simulink model "Project2DigiCont"  (R2017b)
settings: Solver=VariableStepAuto  StartTime=0.0  StopTime=inf  RelTol=1e-3
libraries: Alarm_Library x1, Bump_SensorLib x1, Sensor_Wheellib x1
settings Model: Creator=segadiallo  LastModifiedBy=segadiallo

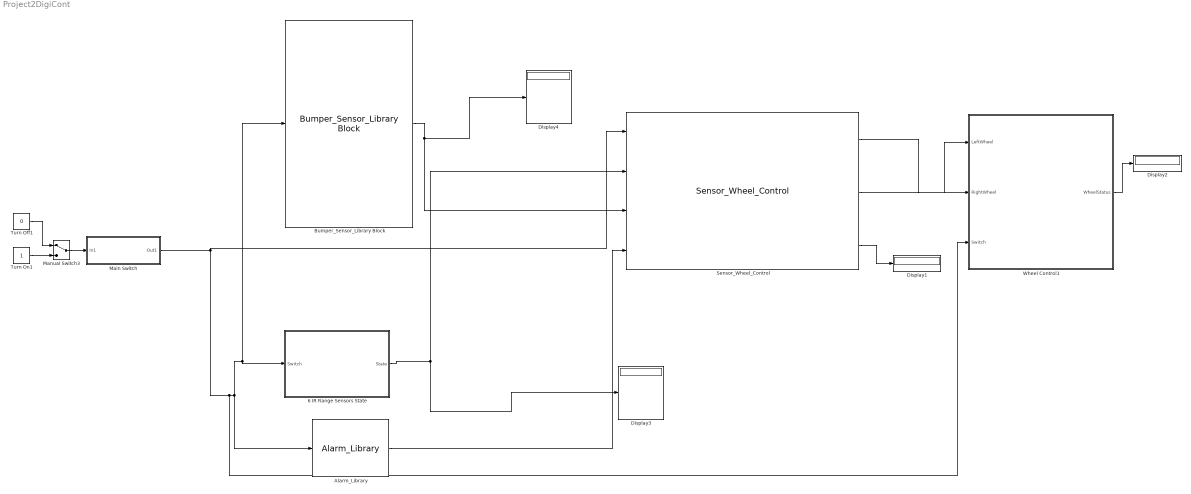
== system Project2DigiCont ==
  6 IR Range Sensors State : Subsystem  AncestorBlock=RoombaSimulink/6 IR Range Sensors State  mask(Sensor Read){}
      mask help:
      | Input 0 to turn off block
      | Input 1 to turn on block
      mask Display:
      | disp('IR Sensors State')
      | port_label('input',1,'Control')
      | port_label('output',1,'State')
  Alarm_Library : Alarm_Library/Alarm_Library  SystemSampleTime=-1
  Bumper_Sensor_Library Block : Bump_SensorLib/Bumper_Sensor_Library Block
  Display{1..4} (4 alike) : Display
  Main Switch : Subsystem
      mask Display:
      | disp('Main Switch')
      | port_label('output',1,'inputV')
      | port_label('input',1,'Go')
  Manual Switch3 : ManualSwitch
  Sensor_Wheel_Control : Sensor_Wheellib/Sensor_Wheel_Control  v0=0.2
  Turn Off1 : Constant  Value=0
  Turn On1 : Constant
  Wheel Control1 : Subsystem  AncestorBlock=RoombaSimulink/Wheel Control  mask(Control){}
      mask help:
      | Input -0.5~0.5 to LeftWheel and RightWheel to control the two wheels independently.
      | Switch: input 0 to turn off block; input 1 to turn on block; input 2 to pause wheel motions.
      mask Display:
      | disp('Wheel Control')
      | port_label('input',1,'LeftWheel')
      | port_label('input',2,'RightWheel')
      | port_label('input',3,'Control')
      | port_label('output',1,'Status')
      | %port_label('input',4,'Break')
  wires:
  Wheel Control1/1(WheelStatus) -> Display2/1
  6 IR Range Sensors State/1("State ") -> Display3/1, Sensor_Wheel_Control/2
  Turn Off1/1 -> Manual Switch3/1
  Turn On1/1 -> Manual Switch3/2
  Manual Switch3/1 -> Main Switch/1(In1)
  Main Switch/1(Out1) -> Wheel Control1/3(Switch), 6 IR Range Sensors State/1(Switch), Bumper_Sensor_Library Block/1, Alarm_Library/1, Sensor_Wheel_Control/1
  Sensor_Wheel_Control/1 -> Wheel Control1/2(RightWheel)
  Sensor_Wheel_Control/2 -> Wheel Control1/1(LeftWheel)
  Bumper_Sensor_Library Block/1 -> Display4/1, Sensor_Wheel_Control/3
  Sensor_Wheel_Control/3 -> Display1/1
  Alarm_Library/1 -> Sensor_Wheel_Control/4

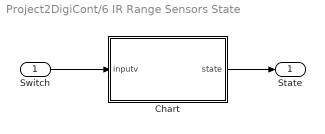
== system Project2DigiCont/6 IR Range Sensors State ==
  Switch : Inport
  Chart : Stateflow chart  TreatAsAtomicUnit=on
  "State " : Outport
  wires:
  Switch/1 -> Chart/1(inputv)
  Chart/1(state) -> "State "/1

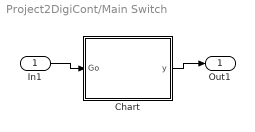
== system Project2DigiCont/Main Switch ==
  In1 : Inport
  Chart : Stateflow chart  TreatAsAtomicUnit=on
  Out1 : Outport
  wires:
  Chart/1(y) -> Out1/1
  In1/1 -> Chart/1(Go)

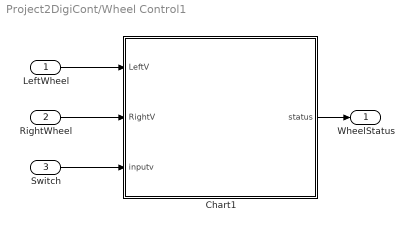
== system Project2DigiCont/Wheel Control1 ==
  LeftWheel : Inport
  RightWheel : Inport  Port=2
  Switch : Inport  Port=3
  Chart1 : Stateflow chart  TreatAsAtomicUnit=on
  WheelStatus : Outport
  wires:
  Switch/1 -> Chart1/3(inputv)
  RightWheel/1 -> Chart1/2(RightV)
  Chart1/1(status) -> WheelStatus/1
  LeftWheel/1 -> Chart1/1(LeftV)

== stateflow chart Project2DigiCont/Wheel Control1/Chart1 ==
  state START
    entry: status=0
  state Connect
    entry: coder.extrinsic('evalin')
    so=evalin('base','objWs')
  state Run
    entry,du:
    coder.extrinsic('SetWheelVelRoomba')
    SetWheelVelRoomba(so,RightV, LeftV)
    status=1
  state Off
    %entry: fclose(so);
    entry:  status=0
  state Pause [commented out]
    entry:
    coder.extrinsic('SetWheelVelRoomba')
    SetWheelVelRoomba(so,0, 0)
    status=2
  (default) -> START
  Off -> Connect : [inputv==4]
  START -> Connect : [inputv==4]
  Connect -> Run [order 2] : [inputv==2]
  Connect -> Off [order 1] : [inputv==0]
  Run -> Off : [inputv==0]
  Pause -> Run [commented out] : [break0==0]
  Run -> Pause [commented out] : [break0==1]
  Pause -> Off [commented out] : [inputv==0]
  data: LeftV input; RightV input; inputv input; status output; so local

== stateflow chart Project2DigiCont/Main Switch/Chart ==
  state START
    entry:
    y=0
  state CONNECT
    entry: tcpInit;
  state DISCONNECT
    entry: y=0
    coder.extrinsic('evalin')
    obj=evalin('base','objWs')
    fclose(obj)
  state Toggle
    entry: y = y + 1
    if y==6
    y=1
    end
  state SerialControl1
    entry: y==1
  (default) -> START
  START -> CONNECT : [Go==1]
  DISCONNECT -> CONNECT : [Go==1]
  CONNECT -> DISCONNECT [order 1] : [Go==0]
  SerialControl1 -> DISCONNECT [order 2] : [Go ==0]
  CONNECT -> SerialControl1 [order 2]
  Toggle -> SerialControl1 : after(1,sec)
  SerialControl1 -> Toggle [order 1] : [Go==1]
  data: Go input; obj local; y output
  function tcpInit:
    | function tcpInit
    | coder.extrinsic('tcpip');
    | coder.extrinsic('assignin');
    | persistent obj
    | 
    | serPort = tcpip('10.0.0.1',9001);
    | set(serPort,'Terminator','LF')
    | set(serPort,'InputBufferSize',1000)
    | set(serPort, 'Timeout', 60)
    | set(serPort, 'ByteOrder','bigEndian');
    | 
    | fopen(serPort);
    | 
    | Start=[128];
    | fwrite(serPort,Start);
    | pause(.1)
    | Mode= 132;
    | fwrite(serPort,Mode);
    | pause(.1)
    | 
    | % %Print 'go' on display
    | fwrite(serPort, [164, 71, 79, 32, 32]);
    | % make a sound
    | fwrite(serPort, [140 1 3 60 20 72 20 84 40 ]); %RoombaInit Song
    | fwrite(serPort, [140 2 1 60 20]); % BeepRoomba song
    | fwrite(serPort, [140 3 3 84 20 72 30 60 40]); % PowerOffRoomba song
    | fwrite(serPort, [141 1]); % play RoombaInit song
    | 
    | obj=serPort;
    | 
    | assignin('base','objWs',obj);
    | end

== stateflow chart Project2DigiCont/6 IR Range Sensors State/Chart ==
  state CONNECT
    entry: coder.extrinsic('evalin')
    so=evalin('base','objWs')
  state START
    entry: state=[0;0;0;0;0;0]
  state READ
    entry,du:
    coder.extrinsic('evalin')
    so=evalin('base','objWs')
    coder.extrinsic('RangeStateRoomba')
    state=RangeStateRoomba(so)
  state TRUNOFF
    %entry: fclose(so)
    entry:  state=[0;0;0;0;0;0]
  (default) -> START
  START -> CONNECT : [inputv==1]
  CONNECT -> READ
  TRUNOFF -> CONNECT : [inputv==1]
  READ -> TRUNOFF : [inputv==0]
  data: state output double size=6; inputv input; so local
